simulink model "lab_03_main"  (R2024b)
settings: Solver=VariableStepAuto  StartTime=0.0  StopTime=10.0  RelTol=1e-3
settings Model: LastModifiedBy=LENOVO

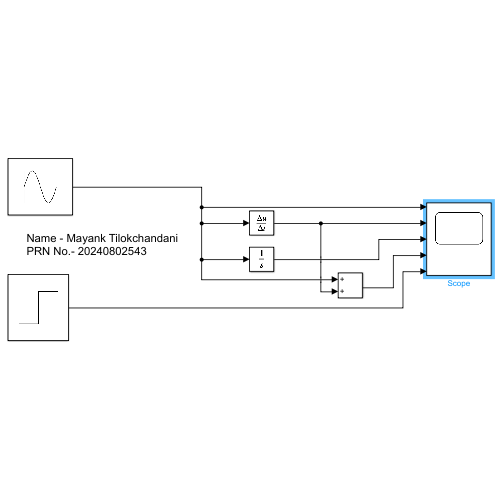
[thumbnail: Simulink's stored preview of the top-level diagram]
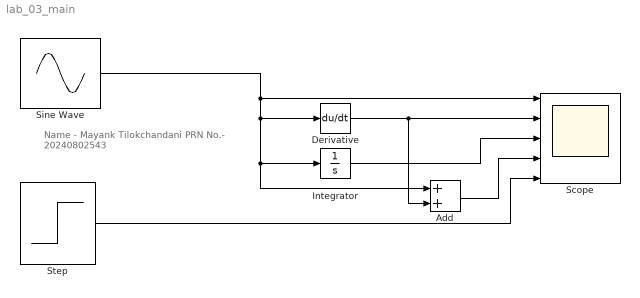
== system lab_03_main ==
  note: Name - Mayank Tilokchandani
      | PRN No.- 20240802543
  Add : Sum
  Derivative : Derivative
  Integrator : Integrator
  Scope : Scope  NumInputPorts=5
  Sine Wave : Sin  SampleTime=0
  Step : Step  SampleTime=0
  wires:
  Add/1 -> Scope/4
  Derivative/1 -> Scope/2, Add/2
  Sine Wave/1 -> Derivative/1, Add/1, Integrator/1, Scope/1
  Integrator/1 -> Scope/3
  Step/1 -> Scope/5
